simulink model "Project1part2c_abhaykela"  (R2014b)
settings: Solver=ode5  StartTime=0.0  StopTime=5  FixedStep=0.01  RelTol=1e-3
settings Model: Creator=axk7578  LastModifiedBy=axk7578

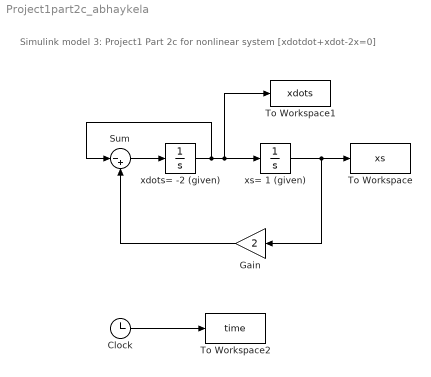
== system Project1part2c_abhaykela ==
  note: Simulink model 3: Project1 Part 2c for nonlinear system [xdotdot+xdot-2x=0]
  Clock : Clock
  Gain : Gain  Gain=2
  Sum : Sum  Inputs=|-+
  To Workspace : ToWorkspace  VariableName=xs  SampleTime=-1
  To Workspace1 : ToWorkspace  VariableName=xdots  SampleTime=-1
  To Workspace2 : ToWorkspace  VariableName=time  SampleTime=-1
  "xdots= -2 (given) " : Integrator  InitialCondition=-2
  xs= 1 (given) : Integrator  InitialCondition=1
  wires:
  xs= 1 (given)/1 -> Gain/1, To Workspace/1
  Sum/1 -> "xdots= -2 (given) "/1
  Clock/1 -> To Workspace2/1
  Gain/1 -> Sum/2
  "xdots= -2 (given) "/1 -> Sum/1, To Workspace1/1, xs= 1 (given)/1
